simulink model "Laboratorio_temperatura"  (R2023a)
settings: Solver=VariableStepAuto  StartTime=0.0  StopTime=6250  RelTol=1e-3  EnableMultiTasking=on
StartFcn:
  | clear all
libraries: realtime_pacer_lib x1, simulink_extras x1
settings Model: Creator=johnh  LastModifiedBy=User
settings SolverCC: AlgebraicLoopSolver=TrustRegion
settings DataIOCC: ReturnWorkspaceOutputs=off
settings OptimizationCC: LifeSpan=inf
settings DebuggingCC: UnconnectedInputMsg=warning  UnconnectedOutputMsg=warning  UnconnectedLineMsg=warning  SFUnexpectedBacktrackingDiag=warning  SFNoUnconditionalDefaultTransitionDiag=warning  SFExecutionAtInitializationDiag=none  ArithmeticOperatorsInVariantConditions=warning
settings ModelReferenceCC: EnableRefExpFcnMdlSchedulingChecks=on
settings SFSimCC: SimUseLocalCustomCode=off  CustomCodeUndefinedFunction=UseInterfaceOnly
settings RTWCC: RTWUseLocalCustomCode=off
settings CodeAppCC: StateflowObjectComments=on
settings GRTTargetCC: TargetLangStandard=C89/C90 (ANSI)
settings ConfigComp: CovMetricSettings=dw  CovSaveCumulativeToWorkspaceVar=on  CovSaveSingleToWorkspaceVar=on  CovExternalEMLEnable=off

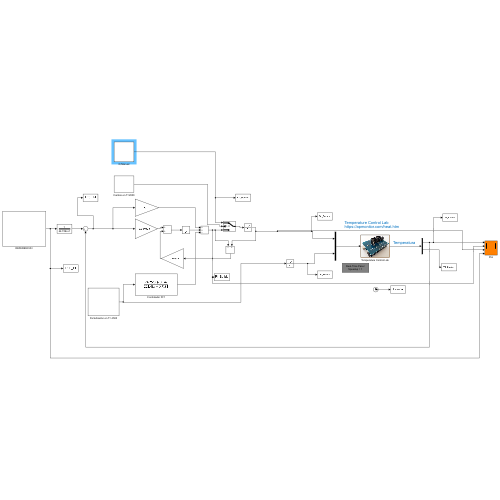
[thumbnail: Simulink's stored preview of the top-level diagram]
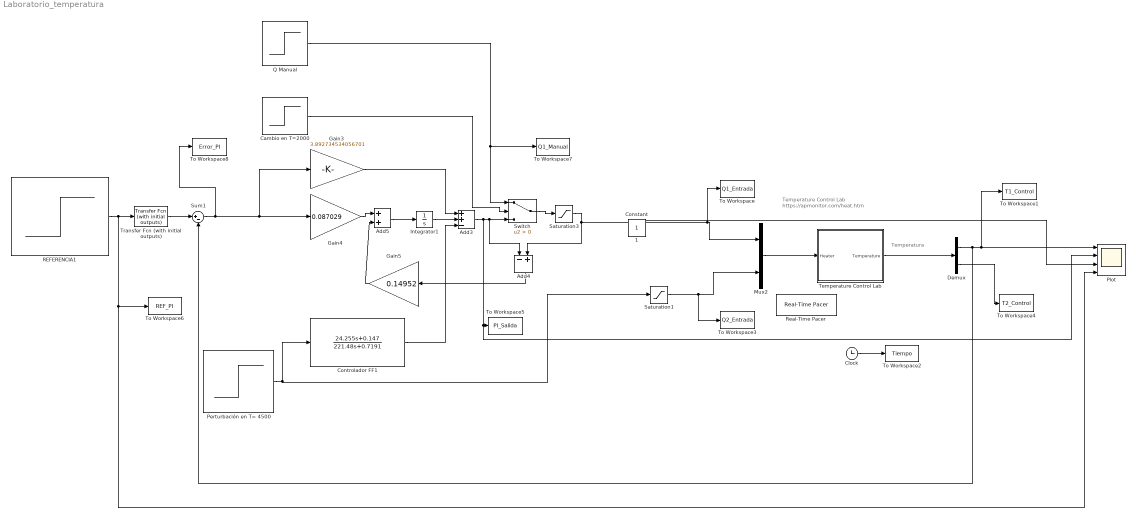
== system Laboratorio_temperatura ==
  note: Temperature Control Lab
      | https://apmonitor.com/heat.htm
  note: Temperatura
  Add3 : Sum  Inputs=++-
  Add4 : Sum  Inputs=-+
  Add5 : Sum
  Cambio en T=2000 : Step  Time=2000  Before=1  After=0  SampleTime=0
  Clock : Clock
  Controlador FF1 : TransferFcn  Numerator=[24.255 0.147]  Denominator=[221.48 0.7191]
  Demux : Demux  Outputs=2
  Gain3 : Gain  Gain=3.892734534056701
  Gain4 : Gain  Gain=0.087029
  Gain5 : Gain  Gain=0.14952
  Integrator1 : Integrator  InitialCondition=13
  Mux2 : Mux  Inputs=2
  Perturbación en T= 4500 : Step  Time=4500  After=20  SampleTime=0
  Plot : Scope  NumInputPorts=4
  Q Manual : Step  After=13  SampleTime=0
  REFERENCIA1 : Step  Time=2000  Before=36.474  After=56.474  SampleTime=0
  Real-Time Pacer : realtime_pacer_lib/Real-Time Pacer  simTimePerRealTime=1
      settings: SourceProductName=Real-Time Pacer
  Saturation1 : Saturate  UpperLimit=100  LowerLimit=0
  Saturation3 : Saturate  UpperLimit=100  LowerLimit=0
  Sum1 : Sum  Inputs=|+-
  Switch : Switch  Criteria=u2 > Threshold  SaturateOnIntegerOverflow=off  InputSameDT=off
  Temperature Control Lab : Subsystem
      mask Display: image('tclab.png');
  To Workspace : ToWorkspace  VariableName=Q1_Entrada  SampleTime=0.5
      settings: Save2DSignal=2-D array (concatenate along first dimension)
  To Workspace1 : ToWorkspace  VariableName=T1_Control  SampleTime=0.5
      settings: Save2DSignal=2-D array (concatenate along first dimension)
  To Workspace2 : ToWorkspace  VariableName=Tiempo  SampleTime=0.5
      settings: Save2DSignal=2-D array (concatenate along first dimension)
  To Workspace3 : ToWorkspace  VariableName=Q2_Entrada  SampleTime=0.5
      settings: Save2DSignal=2-D array (concatenate along first dimension)
  To Workspace4 : ToWorkspace  VariableName=T2_Control  SampleTime=0.5
      settings: Save2DSignal=2-D array (concatenate along first dimension)
  To Workspace5 : ToWorkspace  VariableName=PI_Salida  SampleTime=0.5
      settings: Save2DSignal=2-D array (concatenate along first dimension)
  To Workspace6 : ToWorkspace  VariableName=REF_PI  SampleTime=0.5
      settings: Save2DSignal=2-D array (concatenate along first dimension)
  To Workspace7 : ToWorkspace  VariableName=Q1_Manual  SampleTime=0.5
      settings: Save2DSignal=2-D array (concatenate along first dimension)
  To Workspace8 : ToWorkspace  VariableName=Error_PI  SampleTime=0.5
      settings: Save2DSignal=2-D array (concatenate along first dimension)
  Transfer Fcn (with initial outputs) : simulink_extras/Additional Linear/Transfer Fcn (with initial outputs)  N=[1]  D="[44.729  1]"  Y0=36.47  U0=0
  1 : Constant  IOType=siggen
  Constant : Constant  IOType=siggen
  wires:
  Perturbación en T= 4500/1 -> Controlador FF1/1, Saturation1/1
  Temperature Control Lab/1(Temperature) -> Demux/1
  Mux2/1 -> Temperature Control Lab/1(Heater)
  Demux/2 -> To Workspace4/1
  Demux/1 -> Sum1/2, To Workspace1/1, Plot/1
  Clock/1 -> To Workspace2/1
  Saturation3/1 -> Add4/2, Plot/3, Mux2/1, To Workspace/1
  Saturation1/1 -> To Workspace3/1, Mux2/2
  Add3/1 -> Plot/2, To Workspace5/1, Add4/1, Switch/3
  Integrator1/1 -> Add3/2
  Gain4/1 -> Add5/1
  Add4/1 -> Gain5/1
  Add5/1 -> Integrator1/1
  Gain5/1 -> Add5/2
  Gain3/1 -> Add3/1
  Controlador FF1/1 -> Add3/3
  Sum1/1 -> Gain3/1, Gain4/1, To Workspace8/1
  Switch/1 -> Saturation3/1
  Q Manual/1 -> To Workspace7/1, Switch/1
  Cambio en T=2000/1 -> Switch/2
  Transfer Fcn (with initial outputs)/1 -> Sum1/1
  REFERENCIA1/1 -> Plot/4, To Workspace6/1, Transfer Fcn (with initial outputs)/1

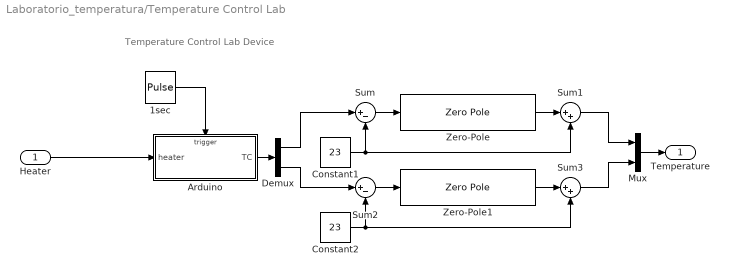
== system Laboratorio_temperatura/Temperature Control Lab ==
  note: Temperature Control Lab Device
  Heater : Inport
  1sec : DiscretePulseGenerator  PulseType=Time based  Period=1  PulseWidth=50
  Arduino : Subsystem  TreatAsAtomicUnit=on
  Constant1 : Constant  Value=23
  Constant2 : Constant  Value=23
  Demux : Demux  Outputs=2
  Mux : Mux  Inputs=2
  Sum : Sum  Inputs=|+-
  Sum1 : Sum  Inputs=|++
  Sum2 : Sum  Inputs=|+-
  Sum3 : Sum  Inputs=|++
  Zero-Pole : ZeroPole  Zeros=[]  Poles=[-0.1 -0.1]  Gain=[0.01]
  Zero-Pole1 : ZeroPole  Zeros=[]  Poles=[-0.1 -0.1]  Gain=[0.01]
  Temperature : Outport  VectorParamsAs1DForOutWhenUnconnected=off
  wires:
  1sec/1 -> Arduino/Trigger
  Heater/1 -> Arduino/1(heater)
  Zero-Pole/1 -> Sum1/1
  Sum2/1 -> Zero-Pole1/1
  Zero-Pole1/1 -> Sum3/1
  Demux/1 -> Sum/1
  Demux/2 -> Sum2/1
  Arduino/1(TC) -> Demux/1
  Constant2/1 -> Sum2/2, Sum3/2
  Mux/1 -> Temperature/1
  Sum3/1 -> Mux/2
  Sum1/1 -> Mux/1
  Constant1/1 -> Sum/2, Sum1/2
  Sum/1 -> Zero-Pole/1

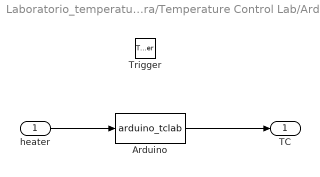
== system Laboratorio_temperatura/Temperature Control Lab/Arduino ==
  heater : Inport  LatchByDelayingOutsideSignal=on
  Trigger : TriggerPort  VariantControl=Variant
  Arduino : MATLABFcn  MATLABFcn=arduino_tclab
  TC : Outport  InitialOutput=[23 23]  VectorParamsAs1DForOutWhenUnconnected=off
  wires:
  heater/1 -> Arduino/1
  Arduino/1 -> TC/1
